simulink model "motore"  (R2024b)
settings: Solver=VariableStepAuto  StartTime=0.0  StopTime=10  RelTol=1e-3
undefined symbols (not defined in the file): Beta, J_macchina, J_motore, kt, kv, La, Ra, Va
settings Model: Creator=USER  LastModifiedBy=USER
settings SolverCC: AlgebraicLoopSolver=TrustRegion
settings DebuggingCC: UnconnectedInputMsg=warning  UnconnectedOutputMsg=warning  UnconnectedLineMsg=warning
settings ModelReferenceCC: EnableRefExpFcnMdlSchedulingChecks=on
settings RTWCC: GPUComputeCapability=3.5  DLArmComputeVersion=19.05

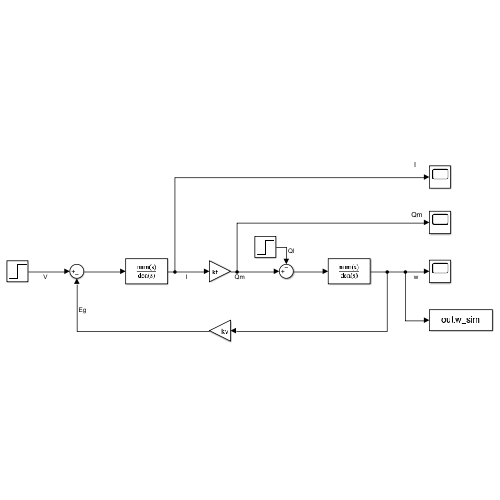
[thumbnail: Simulink's stored preview of the top-level diagram]
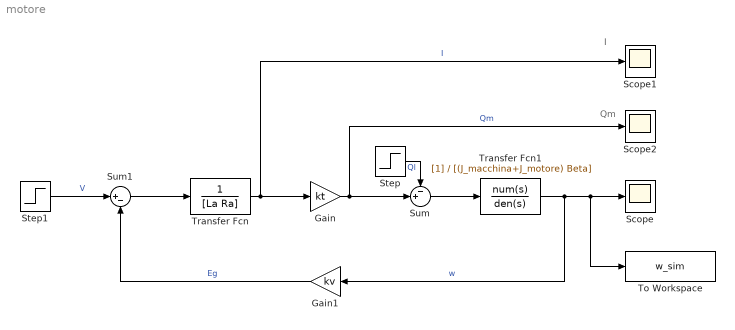
== system motore ==
  note: Qm
  note: I
  Gain : Gain  Gain=kt
  Gain1 : Gain  Gain=kv
  Scope : Scope
  Scope1 : Scope
  Scope2 : Scope
  Step : Step  After=0  SampleTime=0
  Step1 : Step  After=Va  SampleTime=0
  Sum : Sum  Inputs=-+|
  Sum1 : Sum  Inputs=|+-
  To Workspace : ToWorkspace  VariableName=w_sim  SaveFormat=Timeseries  SampleTime=-1
  Transfer Fcn : TransferFcn  Denominator=[La Ra]
  Transfer Fcn1 : TransferFcn  Denominator=[(J_macchina+J_motore) Beta]
  wires:
  Transfer Fcn/1 -> Scope1/1, Gain/1  "I"
  Gain/1 -> Sum/2, Scope2/1  "Qm"
  Sum/1 -> Transfer Fcn1/1
  Step/1 -> Sum/1  "Ql"
  Transfer Fcn1/1 -> Gain1/1, To Workspace/1, Scope/1  "w"
  Gain1/1 -> Sum1/2  "Eg"
  Sum1/1 -> Transfer Fcn/1
  Step1/1 -> Sum1/1  "V"
